simulink model "BACKUP"  (R2023a)
settings: Solver=VariableStepAuto  StartTime=0.0  StopTime=10.0  RelTol=1e-3
undefined symbols (not defined in the file or in its folder): q_0, qdot_0
settings Model: Creator=dervint  LastModifiedBy=dervint

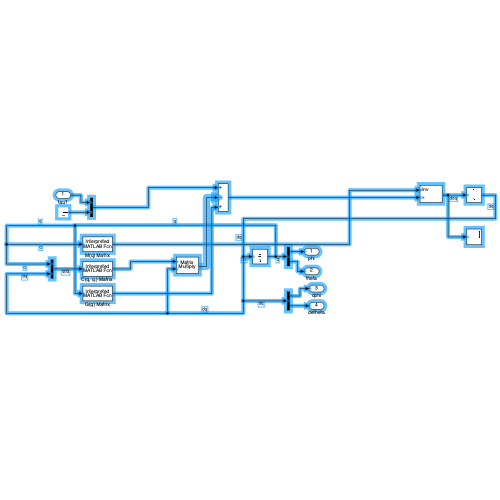
[thumbnail: Simulink's stored preview of the top-level diagram]
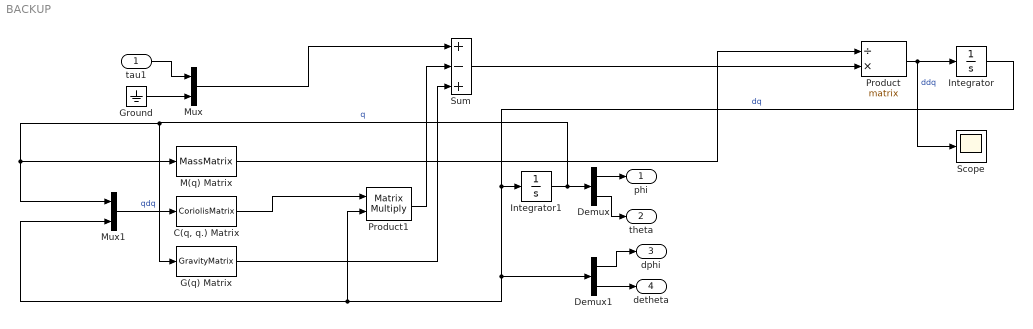
== system BACKUP ==
  tau1 : Inport
  "C(q, q.) Matrix " : MATLABFcn  MATLABFcn=CoriolisMatrix  Output1D=off
  Demux : Demux  Outputs=2
  Demux1 : Demux  Outputs=2
  G(q) Matrix : MATLABFcn  MATLABFcn=GravityMatrix
  Ground : Ground
  Integrator : Integrator  InitialCondition=qdot_0
  Integrator1 : Integrator  InitialCondition=q_0
  M(q) Matrix : MATLABFcn  MATLABFcn=MassMatrix  Output1D=off
  Mux : Mux  Inputs=2
  Mux1 : Mux  Inputs=2
  Product : Product  Inputs=/*  Multiplication=Matrix(*)  InputSameDT=on  SaturateOnIntegerOverflow=on  OutDataTypeStr=Inherit: Same as first input
  Product1 : Product  Multiplication=Matrix(*)  InputSameDT=on  SaturateOnIntegerOverflow=on  OutDataTypeStr=Inherit: Same as first input
  Scope : Scope
  Sum : Sum  Inputs=+-+  InputSameDT=on  SaturateOnIntegerOverflow=on  OutDataTypeStr=Inherit: Same as first input
  phi : Outport
  theta : Outport  Port=2
  dphi : Outport  Port=3
  detheta : Outport  Port=4
  wires:
  Product/1 -> Scope/1, Integrator/1  "ddq"
  Demux1/1 -> dphi/1
  Demux1/2 -> detheta/1
  tau1/1 -> Mux/1
  Ground/1 -> Mux/2
  Mux/1 -> Sum/1
  Integrator1/1 -> Mux1/1, M(q) Matrix/1, G(q) Matrix/1, Demux/1  "q"
  "C(q, q.) Matrix "/1 -> Product1/1
  Demux/2 -> theta/1
  Demux/1 -> phi/1
  Integrator/1 -> Demux1/1, Mux1/2, Product1/2, Integrator1/1  "dq"
  M(q) Matrix/1 -> Product/1
  Mux1/1 -> "C(q, q.) Matrix "/1  "qdq"
  Sum/1 -> Product/2
  G(q) Matrix/1 -> Sum/3
  Product1/1 -> Sum/2
